simulink model "CL_linear_mdl_with_State_Feedback"  (R2024b)
settings: Solver=FixedStepAuto  StartTime=0.0  StopTime=Tsim  FixedStep=1e-7  RelTol=1e-3
values from neighbouring files (symbols this model uses):
  K = lqr(plant_ss.A, plant_ss.B, Q, R)    [Copy_of_main_final.m]    (also in test_anime.m = lqr(A, B, Q, Rw))
  plant_ss = plant_ss_q1    [Copy_of_main_final.m]    (also in syst_repr_generator.m = ss(A,B,C,D))
  q20 = 10    [Copy_of_main_final.m]
settings Model: Creator=dsagn  LastModifiedBy=dsagn
settings SolverCC: AlgebraicLoopSolver=TrustRegion
settings DataIOCC: ReturnWorkspaceOutputs=off
settings DebuggingCC: UnconnectedInputMsg=warning  UnconnectedOutputMsg=warning  UnconnectedLineMsg=warning  ArithmeticOperatorsInVariantConditions=warning
settings ModelReferenceCC: EnableRefExpFcnMdlSchedulingChecks=on
settings SFSimCC: CustomCodeUndefinedFunction=UseInterfaceOnly
settings RTWCC: GPUComputeCapability=3.5

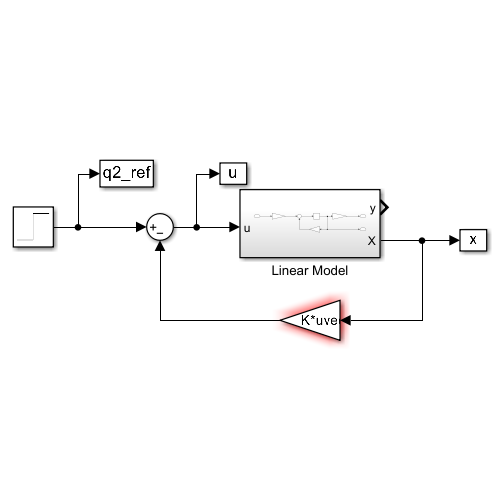
[thumbnail: Simulink's stored preview of the top-level diagram]
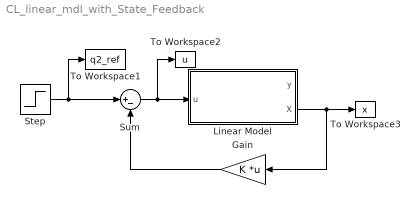
== system CL_linear_mdl_with_State_Feedback ==
  Gain : Gain  Gain=K  Multiplication=Matrix(K*u) (u vector)
  Linear Model : Subsystem
  Step : Step  After=0  SampleTime=0
  Sum : Sum  Inputs=|+-
  To Workspace1 : ToWorkspace  VariableName=q2_ref  SaveFormat=Timeseries  SampleTime=-1
  To Workspace2 : ToWorkspace  VariableName=u  SaveFormat=Timeseries  SampleTime=-1
  To Workspace3 : ToWorkspace  VariableName=x  SaveFormat=Timeseries  SampleTime=-1
  wires:
  Step/1 -> Sum/1, To Workspace1/1
  Sum/1 -> To Workspace2/1, Linear Model/1(u)
  Linear Model/2(X) -> Gain/1, To Workspace3/1
  Gain/1 -> Sum/2

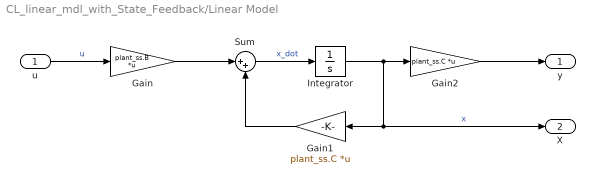
== system CL_linear_mdl_with_State_Feedback/Linear Model ==
  u : Inport
  Gain : Gain  Gain=plant_ss.B  Multiplication=Matrix(K*u) (u vector)
  Gain1 : Gain  Gain=plant_ss.C  Multiplication=Matrix(K*u) (u vector)
  Gain2 : Gain  Gain=plant_ss.C  Multiplication=Matrix(K*u) (u vector)
  Integrator : Integrator  InitialCondition=[0,q20,0,0]
  Sum : Sum  Inputs=|++
  y : Outport  VectorParamsAs1DForOutWhenUnconnected=off
  X : Outport  Port=2
  wires:
  Gain/1 -> Sum/1
  Integrator/1 -> X/1, Gain1/1, Gain2/1  "x"
  Sum/1 -> Integrator/1  "x_dot"
  Gain1/1 -> Sum/2
  u/1 -> Gain/1  "u"
  Gain2/1 -> y/1
